simulink model "pmsm_detailed_drive"  (R2014a)
settings: Solver=FixedStepDiscrete  SolverMode=SingleTasking  StartTime=0.0  StopTime=4  FixedStep=Ts  RelTol=1e-4
PreLoadFcn:
  | Ts=1e-5;
  | Tc=4e-4;
StartFcn:
  | tic;
StopFcn:
  | toc;
libraries: powerlib x9, powerlib_meascontrol x5, simulink x3
Description:
  | Copyright 2008 The MathWorks(TM), Inc.
settings Model: ExtModeTrigMode=oneshot  ExtModeArmWhenConnect=off  ExtModeAutoUpdateStatusClock=off  Creator=patrice  LastModifiedBy=cosorio
settings DataIOCC: ExternalInput=[]  LimitDataPoints=off  SignalLoggingSaveFormat=ModelDataLogs  SaveOutput=off  SaveTime=off  SignalLoggingName=sigsOut
settings OptimizationCC: BlockReduction=off  BooleanDataType=off  ExpressionDepthLimit=2147483647  InitFltsAndDblsToZero=on  EfficientMapNaN2IntZero=off
settings DebuggingCC: UnderspecifiedInitializationDetection=Classic  CheckExecutionContextPreStartOutputMsg=on  CheckExecutionContextRuntimeOutputMsg=on  SignalResolutionControl=TryResolveAllWithWarning  SolverPrmCheckMsg=none  MultiTaskDSMMsg=warning  MultiTaskCondExecSysMsg=none  SigSpecEnsureSampleTimeMsg=none  FcnCallInpInsideContextMsg=UseLocalSettings  StateNameClashWarn=warning
settings HardwareCC: TargetUnknown=on
settings RTWCC: IncludeERTFirstTime=on
settings GRTTargetCC: CombineOutputUpdateFcns=off  GRTInterface=on

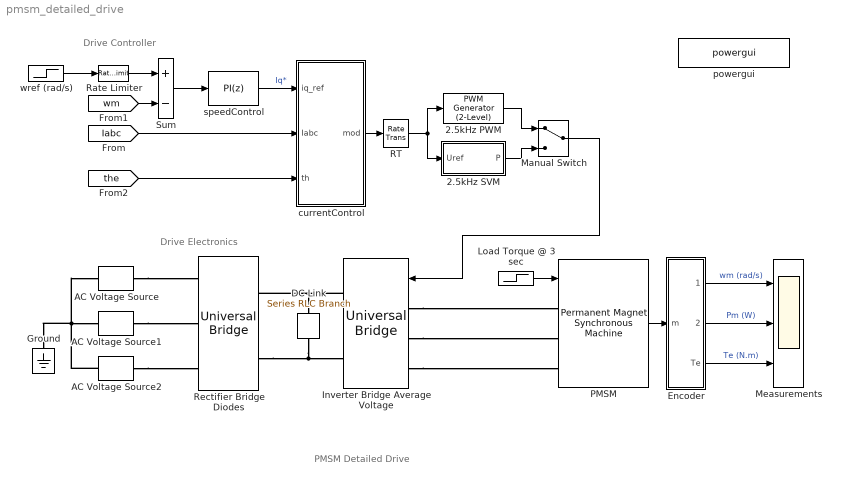
== system pmsm_detailed_drive ==
  note: Drive Controller
  note: PMSM Detailed Drive
  note: Drive Electronics
  2.5kHz PWM : powerlib_meascontrol/Pulse & Signal Generators/PWM Generator (2-Level)  ModulatorType=Three-phase bridge (6 pulses)  ModulatorMode=Unsynchronized  nF=27  Fc=1/Tc  ModulatingSignals=off  m=0.8  Freq=60  Phase=0  Ts=Ts
  2.5kHz SVM : Subsystem
  AC Voltage Source : powerlib/Electrical Sources/AC Voltage Source  Amplitude=600*sqrt(2)/sqrt(3)  Phase=30  Frequency=60  SampleTime=Ts  Measurements=None
  AC Voltage Source1 : powerlib/Electrical Sources/AC Voltage Source  Amplitude=600*sqrt(2)/sqrt(3)  Phase=-120+30  Frequency=60  SampleTime=Ts  Measurements=None
  AC Voltage Source2 : powerlib/Electrical Sources/AC Voltage Source  Amplitude=600*sqrt(2)/sqrt(3)  Phase=120+30  Frequency=60  SampleTime=Ts  Measurements=None
  DC Link : powerlib/Elements/Series RLC Branch  LConnTagsString=__new0  RConnTagsString=__new0  BranchType=C  Resistance=1  Inductance=1e-3  SetiL0=off  InitialCurrent=0  Capacitance=3600e-6  Setx0=off  InitialVoltage=0  Measurements=None
  Encoder : Subsystem
  Ground : powerlib/Elements/Ground  LConnTagsString=a
  Inverter Bridge Average Voltage : powerlib/Power Electronics/Universal Bridge  Arms=3  SnubberResistance=1e4  SnubberCapacitance=1e-5  Device=IGBT / Diodes  Ron=1e-4  Lon=0  ForwardVoltages="[  0  0  ]"  ForwardVoltage=0  GTOparameters=[ 10e-6 , 20e-6 ]  IGBTparameters=[ 1e-6 , 2e-6 ]  Measurements=None  Measurements_2=None  converterType=Rectifier
  Load Torque @ 3 sec : Step  Time=3  Before=10  After=20  SampleTime=Ts
  Manual Switch : ManualSwitch
  Measurements : Scope  NumInputPorts=3
      settings: YMin=0~0~0  YMax=250~15000~80  SaveName=PMSMData  SampleTime=Ts
  PMSM : powerlib/Machines/Permanent Magnet Synchronous Machine  NbPhases=3  FluxDistribution=Sinusoidal  RotorType=Salient-pole  MechanicalLoad=Torque Tm  PresetModel=No  ShowDetailedParameters=on  MeasurementBus=off  Resistance=2.875/10  Inductance=8.5e-3  dqInductances=[8.5e-3, 8.5e-3]  La=0.000835  MachineConstant=Flux linkage established by magnets (V.s)  Flux=0.175  VoltageCst=126.966  TorqueCst=1.05  Flat=0  Mechanical="[ 0.5, 0,  4 ]"  PolePairs=4  InitialConditions=[0,0, 0,0]  InitialConditions5ph=[0 0 0 0 0 0]  TsPowergui=0  TsBlock=-1  RefAngle=90 degrees behind phase A axis (modified Park)
      settings: AttributesFormatString=\n
  RT : RateTransition
  Rate Limiter : RateLimiter  RisingSlewLimit=100  FallingSlewLimit=-100  SampleTimeMode=inherited
  Rectifier Bridge Diodes : powerlib/Power Electronics/Universal Bridge  Arms=3  SnubberResistance=1e4  SnubberCapacitance=1e-5  Device=Diodes  Ron=1e-4  Lon=0  ForwardVoltages="[  0  0  ]"  ForwardVoltage=0  GTOparameters=[ 10e-6 , 20e-6 ]  IGBTparameters=[ 1e-6 , 2e-6 ]  Measurements=None  Measurements_2=None  converterType=Rectifier
  Sum : Sum  Inputs=+-  SaturateOnIntegerOverflow=on  InputSameDT=on  OutDataTypeStr=Inherit: Same as first input
  currentControl : Subsystem
  powergui : powerlib/powergui  SimulationMode=Discrete  SolverType=Tustin  SampleTime=Ts  frequency=60  SPID=off  DisableSnubberDevices=off  DisableRonSwitches=off  DisableVfSwitches=off  SwTol=0  Interpol=off  DisplayEquations=off  Ts=0  methode=off  frequencyindice=0  Pbase=100e6  ErrMax=1e-4  Iterations=50  UnitsV=kV  UnitsW=MW  FunctionMessages=off  echomessages=off  HookPort=off  EnableUseOfTLC=off  x0status=blocks  RestoreLinks=warning  ResistiveCurrentMeasurement=off  Frange=[0:2:500]  Ylog=off  Xlog=on  ShowGrid=off  save=off  variable=ZData  structure=Vmod  ZoomFFT=on  StartTime=2.4  cycles=10  DisplayStyle=1  fundamental=100  FreqAxis=on  MaxFrequency=6500  frequencyindicesteady=1  RmsSteady=1  display=off
  speedControl : simulink/Continuous/PID Controller  Controller=PI  TimeDomain=Discrete-time  SampleTime=Tc  IntegratorMethod=Forward Euler  FilterMethod=Forward Euler  Form=Parallel  P=20  I=10  D=0  N=100  InitialConditionSource=internal  InitialConditionForIntegrator=0  InitialConditionForFilter=0  ExternalReset=none  LimitOutput=on  UpperSaturationLimit=200  LowerSaturationLimit=-200  LinearizeAsGain=off  AntiWindupMode=none  Kb=1  TrackingMode=off  Kt=1  PParamMin=[]  PParamMax=[]  IParamMin=[]  IParamMax=[]  DParamMin=[]  DParamMax=[]  NParamMin=[]  NParamMax=[]  KbParamMin=[]  KbParamMax=[]  KtParamMin=[]  KtParamMax=[]  POutMin=[]  POutMax=[]  IOutMin=[]  IOutMax=[]  DOutMin=[]  DOutMax=[]  NOutMin=[]  NOutMax=[]  KbOutMin=[]  KbOutMax=[]  KtOutMin=[]  KtOutMax=[]  IntegratorOutMin=[]  IntegratorOutMax=[]  FilterOutMin=[]  FilterOutMax=[]  SumOutMin=[]  SumOutMax=[]  SumI1OutMin=[]  SumI1OutMax=[]  SumI2OutMin=[]  SumI2OutMax=[]  SumI3OutMin=[]  SumI3OutMax=[]  SumDOutMin=[]  SumDOutMax=[]  SaturationOutMin=[]  SaturationOutMax=[]  IntegratorContinuousStateAttributes=''  IntegratorStateMustResolveToSignalObject=off  IntegratorRTWStateStorageClass=Auto  FilterContinuousStateAttributes=''  FilterStateMustResolveToSignalObject=off  FilterRTWStateStorageClass=Auto
  wref (rad/s) : Step  Time=0  After=200  SampleTime=Tc
  wires:
  Sum/1 -> speedControl/1
  wref (rad/s)/1 -> Rate Limiter/1
  Load Torque @ 3 sec/1 -> PMSM/1
  speedControl/1 -> currentControl/1(iq_ref)  "Iq*"
  [wm] -> Sum/2
  PMSM/1 -> Encoder/1(m)
  Encoder/1(wm) -> Measurements/1  "wm (rad/s)"
  Encoder/2(Pm) -> Measurements/2  "Pm (W)"
  Encoder/3(Te) -> Measurements/3  "Te (N.m)"
  [Iabc] -> currentControl/2(Iabc)
  [the] -> currentControl/3(th)
  currentControl/1(mod) -> RT/1
  2.5kHz PWM/1 -> Manual Switch/1
  Manual Switch/1 -> Inverter Bridge Average Voltage/1
  2.5kHz SVM/1(P) -> Manual Switch/2
  RT/1 -> 2.5kHz PWM/1, 2.5kHz SVM/1(Uref)
  Rate Limiter/1 -> Sum/1
  connections:
  Rectifier Bridge Diodes/RConn2 -- DC Link/RConn1 -- Inverter Bridge Average Voltage/RConn2
  AC Voltage Source2/LConn1 -- AC Voltage Source1/LConn1 -- AC Voltage Source/LConn1 -- Ground/LConn1
  AC Voltage Source2/RConn1 -- Rectifier Bridge Diodes/LConn3
  AC Voltage Source/RConn1 -- Rectifier Bridge Diodes/LConn1
  AC Voltage Source1/RConn1 -- Rectifier Bridge Diodes/LConn2
  Inverter Bridge Average Voltage/RConn1 -- DC Link/LConn1 -- Rectifier Bridge Diodes/RConn1
  Inverter Bridge Average Voltage/LConn1 -- PMSM/LConn1
  Inverter Bridge Average Voltage/LConn2 -- PMSM/LConn2
  Inverter Bridge Average Voltage/LConn3 -- PMSM/LConn3

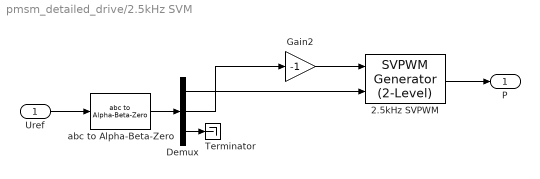
== system pmsm_detailed_drive/2.5kHz SVM ==
  Uref : Inport
  2.5kHz SVPWM : powerlib_meascontrol/Pulse & Signal Generators/SVPWM Generator (2-Level)  InputType=alpha-beta components  SwitchingPattern=Pattern #1  Fc=1/Tc  ParUref=[0.8 -30 50]  Ts=Ts
  Demux : Demux  Outputs=3
  Gain2 : Gain  Gain=-1
  Terminator : Terminator
  abc to Alpha-Beta-Zero : powerlib_meascontrol/Transformations/abc to Alpha-Beta-Zero
  P : Outport
  wires:
  Uref/1 -> abc to Alpha-Beta-Zero/1
  abc to Alpha-Beta-Zero/1 -> Demux/1
  Demux/1 -> 2.5kHz SVPWM/2
  Demux/2 -> Gain2/1
  Demux/3 -> Terminator/1
  2.5kHz SVPWM/1 -> P/1
  Gain2/1 -> 2.5kHz SVPWM/1

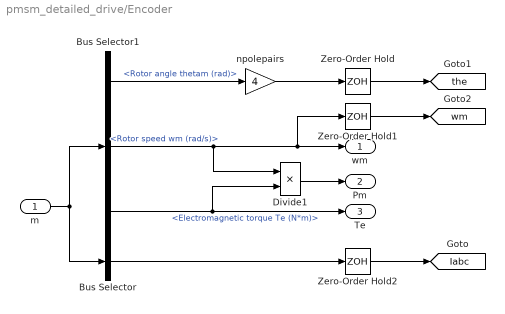
== system pmsm_detailed_drive/Encoder ==
  m : Inport
  Bus Selector : BusSelector  OutputSignals=Stator current is_a (A),Stator current is_b (A),Stator current is_c (A)  OutputAsBus=on
  Bus Selector1 : BusSelector  OutputSignals=Rotor angle thetam (rad),Rotor speed wm (rad/s),Electromagnetic torque Te (N*m)
  Divide1 : Product  Inputs=**
  Zero-Order Hold : ZeroOrderHold  SampleTime=Tc
  Zero-Order Hold1 : ZeroOrderHold  SampleTime=Tc
  Zero-Order Hold2 : ZeroOrderHold  SampleTime=Tc
  "npolepairs " : Gain  Gain=4  SaturateOnIntegerOverflow=on  OutDataTypeStr=Inherit: Same as input  ParamDataTypeStr=Inherit: Same as input
  wm : Outport
  Pm : Outport  Port=2
  Te : Outport  Port=3
  tag scope: Iabc=global, the=global, wm=global
  wires:
  Bus Selector1/3 -> Divide1/2, Te/1  "<Electromagnetic torque Te (N*m)>"
  Bus Selector/1 -> Zero-Order Hold2/1
  Bus Selector1/2 -> Zero-Order Hold1/1, wm/1, Divide1/1  "<Rotor speed wm (rad/s)>"
  Bus Selector1/1 -> "npolepairs "/1  "<Rotor angle thetam (rad)>"
  m/1 -> Bus Selector/1, Bus Selector1/1
  "npolepairs "/1 -> Zero-Order Hold/1
  Divide1/1 -> Pm/1
  Zero-Order Hold/1 -> [the]
  Zero-Order Hold1/1 -> [wm]
  Zero-Order Hold2/1 -> [Iabc]

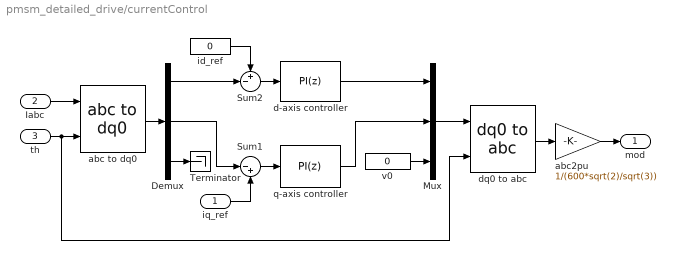
== system pmsm_detailed_drive/currentControl ==
  iq_ref : Inport
  Iabc : Inport  Port=2
  th : Inport  Port=3
  Demux : Demux  Outputs=3
  Mux : Mux  Inputs=3
  Sum1 : Sum  Inputs=|-+
  Sum2 : Sum  Inputs=+-|
  Terminator : Terminator
  abc to dq0 : powerlib_meascontrol/Transformations/abc to dq0  Alignment=90 degrees behind phase A axis
  abc2pu : Gain  Gain=1/(600*sqrt(2)/sqrt(3))
  d-axis controller : simulink/Continuous/PID Controller  Controller=PI  TimeDomain=Discrete-time  SampleTime=Tc  IntegratorMethod=Forward Euler  FilterMethod=Forward Euler  Form=Parallel  P=10  I=100  D=0  N=100  InitialConditionSource=internal  InitialConditionForIntegrator=0  InitialConditionForFilter=0  ExternalReset=none  LimitOutput=on  UpperSaturationLimit=800  LowerSaturationLimit=-800  LinearizeAsGain=off  AntiWindupMode=none  Kb=1  TrackingMode=off  Kt=1  PParamMin=[]  PParamMax=[]  IParamMin=[]  IParamMax=[]  DParamMin=[]  DParamMax=[]  NParamMin=[]  NParamMax=[]  KbParamMin=[]  KbParamMax=[]  KtParamMin=[]  KtParamMax=[]  POutMin=[]  POutMax=[]  IOutMin=[]  IOutMax=[]  DOutMin=[]  DOutMax=[]  NOutMin=[]  NOutMax=[]  KbOutMin=[]  KbOutMax=[]  KtOutMin=[]  KtOutMax=[]  IntegratorOutMin=[]  IntegratorOutMax=[]  FilterOutMin=[]  FilterOutMax=[]  SumOutMin=[]  SumOutMax=[]  SumI1OutMin=[]  SumI1OutMax=[]  SumI2OutMin=[]  SumI2OutMax=[]  SumI3OutMin=[]  SumI3OutMax=[]  SumDOutMin=[]  SumDOutMax=[]  SaturationOutMin=[]  SaturationOutMax=[]  IntegratorContinuousStateAttributes=''  IntegratorStateMustResolveToSignalObject=off  IntegratorRTWStateStorageClass=Auto  FilterContinuousStateAttributes=''  FilterStateMustResolveToSignalObject=off  FilterRTWStateStorageClass=Auto
  dq0 to abc : powerlib_meascontrol/Transformations/dq0 to abc  Alignment=90 degrees behind phase A axis
  id_ref : Constant  Value=0  SampleTime=Tc
  q-axis controller : simulink/Continuous/PID Controller  Controller=PI  TimeDomain=Discrete-time  SampleTime=Tc  IntegratorMethod=Forward Euler  FilterMethod=Forward Euler  Form=Parallel  P=10  I=100  D=0  N=100  InitialConditionSource=internal  InitialConditionForIntegrator=0  InitialConditionForFilter=0  ExternalReset=none  LimitOutput=on  UpperSaturationLimit=800  LowerSaturationLimit=-800  LinearizeAsGain=off  AntiWindupMode=none  Kb=1  TrackingMode=off  Kt=1  PParamMin=[]  PParamMax=[]  IParamMin=[]  IParamMax=[]  DParamMin=[]  DParamMax=[]  NParamMin=[]  NParamMax=[]  KbParamMin=[]  KbParamMax=[]  KtParamMin=[]  KtParamMax=[]  POutMin=[]  POutMax=[]  IOutMin=[]  IOutMax=[]  DOutMin=[]  DOutMax=[]  NOutMin=[]  NOutMax=[]  KbOutMin=[]  KbOutMax=[]  KtOutMin=[]  KtOutMax=[]  IntegratorOutMin=[]  IntegratorOutMax=[]  FilterOutMin=[]  FilterOutMax=[]  SumOutMin=[]  SumOutMax=[]  SumI1OutMin=[]  SumI1OutMax=[]  SumI2OutMin=[]  SumI2OutMax=[]  SumI3OutMin=[]  SumI3OutMax=[]  SumDOutMin=[]  SumDOutMax=[]  SaturationOutMin=[]  SaturationOutMax=[]  IntegratorContinuousStateAttributes=''  IntegratorStateMustResolveToSignalObject=off  IntegratorRTWStateStorageClass=Auto  FilterContinuousStateAttributes=''  FilterStateMustResolveToSignalObject=off  FilterRTWStateStorageClass=Auto
  v0 : Constant  Value=0  SampleTime=Tc
  mod : Outport
  wires:
  Sum1/1 -> q-axis controller/1
  q-axis controller/1 -> Mux/2
  v0/1 -> Mux/3
  d-axis controller/1 -> Mux/1
  Sum2/1 -> d-axis controller/1
  dq0 to abc/1 -> abc2pu/1
  iq_ref/1 -> Sum1/2
  th/1 -> abc to dq0/2, dq0 to abc/2
  Iabc/1 -> abc to dq0/1
  id_ref/1 -> Sum2/1
  abc to dq0/1 -> Demux/1
  Demux/1 -> Sum2/2
  Demux/2 -> Sum1/1
  Demux/3 -> Terminator/1
  abc2pu/1 -> mod/1
  Mux/1 -> dq0 to abc/1
